simulink model "Exercises_lesson_II"  (R2022b)
settings: Solver=ode23tb  StartTime=0.0  StopTime=10  RelTol=1e-3
values from neighbouring files (symbols this model uses):
  Kb = (ki/kp)    (= 0.25)    [PI_par.m]
  ki = wc * Ri    (= 0.125)    [PI_par.m]
  kp = wc * Li    (= 0.5)    [PI_par.m]
  Li = 0.1    [PI_par.m]
  Ri = 0.025    [PI_par.m]
  sat = 0.3    [PI_par.m]
undefined symbols (not defined in the file or in its folder): sigbuilder_block
libraries: slpidlib x3, spsControlledVoltageSourceLib x1, spsCurrentMeasurementLib x1, spsSeriesRLCBranchLib x1, sps_lib x1
settings Model: Creator=matti  LastModifiedBy=benve
settings SolverCC: AlgebraicLoopSolver=TrustRegion
settings DataIOCC: ReturnWorkspaceOutputs=off
settings DebuggingCC: UnconnectedInputMsg=warning  UnconnectedOutputMsg=warning  UnconnectedLineMsg=warning  SFMachineParentedDataDiag=warning  ArithmeticOperatorsInVariantConditions=warning
settings ModelReferenceCC: EnableRefExpFcnMdlSchedulingChecks=on
settings SFSimCC: SimUseLocalCustomCode=off  CustomCodeUndefinedFunction=UseInterfaceOnly
settings RTWCC: RTWUseLocalCustomCode=off
settings CodeAppCC: StateflowObjectComments=on

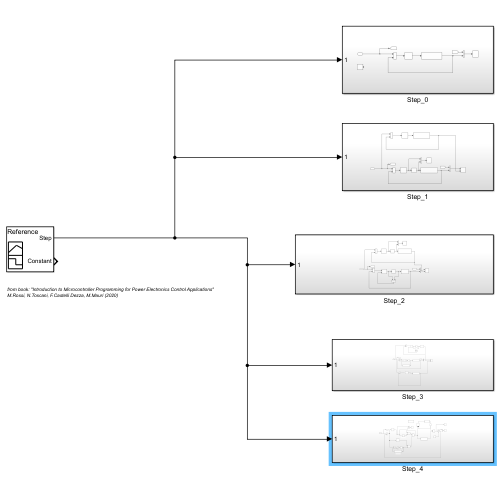
[thumbnail: Simulink's stored preview of the top-level diagram]
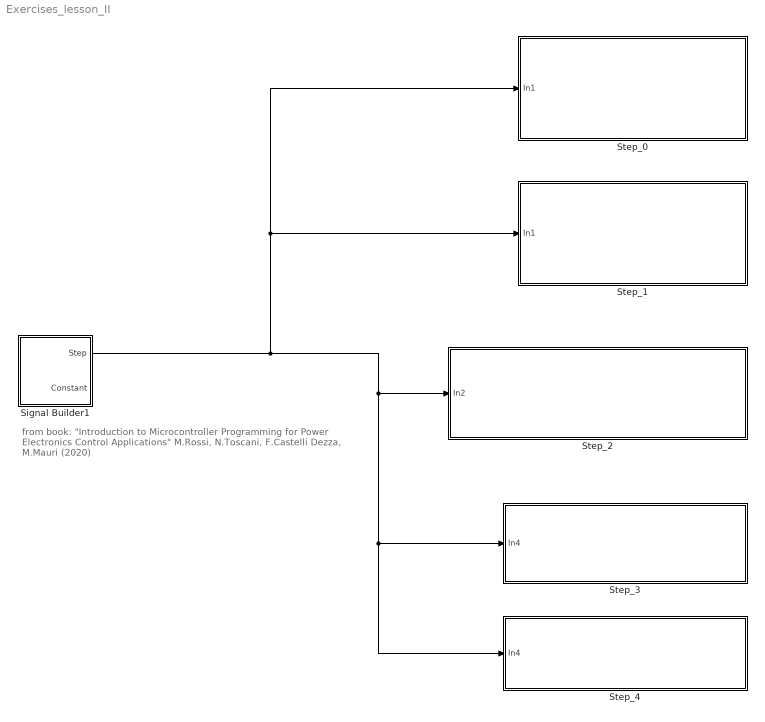
== system Exercises_lesson_II ==
  note: from book: "Introduction to Microcontroller Programming for Power Electronics Control Applications"
      | M.Rossi, N.Toscani, F.Castelli Dezza, M.Mauri (2020)
  Signal Builder1 : Subsystem  Tag=STV Subsys  LoadFcn=sigbuilder_block('load');  StartFcn=sigbuilder_block('start');  StopFcn=sigbuilder_block('stop');  ClipboardFcn=sigbuilder_block('clipboard');  mask(Sigbuilder block){tuvar=[0:10]}
      mask help: Simulink:masks:SigbuilderBlock_MD
      mask init:
      | if ~strcmp(get_param(bdroot(gcbh),'SimulationStatus'),'stopped') tuvar = sigbuilder_block('maskInit'); end
      settings: CopyFcn=sigbuilder_block('copy');  DeleteFcn=sigbuilder_block('delete');  ModelCloseFcn=sigbuilder_block('modelClose');  PreSaveFcn=sigbuilder_block('preSave');  PauseFcn=sigbuilder_block('pause');  ContinueFcn=sigbuilder_block('continue');  NameChangeFcn=sigbuilder_block('namechange');  OpenFcn=sigbuilder_block('open',[5.4 5.4 1141.2 580.8 ]);  CloseFcn=sigbuilder_block('close');
      mask Display: plot(0, 0, 100, 100,[2, 2, 32, 32, 2], [68, 8, 8, 68, 68],[32, 2], [38, 38], [32, 19, 2],[53, 60, 44], [32, 17, 17, 2],[16, 16, 31, 31]);txt = getActiveGroup(gcbh);text(2, 100, txt,'verticalAlignment', 'top');
  Step_0 : Subsystem
  Step_1 : Subsystem
  Step_2 : Subsystem
  Step_3 : Subsystem
  Step_4 : Subsystem
  wires:
  Signal Builder1/1(Step) -> Step_4/1(In4), Step_3/1(In4), Step_2/1(In2), Step_0/1(In1), Step_1/1(In1)

== system Exercises_lesson_II/Signal Builder1 ==
  Demux : Demux  Tag=STV Demux  Outputs=2
      settings: DisplayOption=none
  FromWs : FromWorkspace  Tag=STV FromWs  VariableName=tuvar
      SigBuilderData=|
      | common.afterFinalStr = 'Extrapolate'
      | common.sampleTime = 0
      | dataSet.timeRange = [0 10]
      | dataSet.name = 'Reference'
      | sbobj.Groups.Name = 'Reference'
      | sbobj.Groups.Signals(1).Name = 'Step'
      | sbobj.Groups.Signals(1).XData = [0 1 1 4 4 10]
      | sbobj.Groups.Signals(1).YData = [0 0 1 1 0 0]
      | sbobj.Groups.Signals(2).Name = 'Constant'
      | sbobj.Groups.Signals(2).XData = [0 10]
      | sbobj.Groups.Signals(2).YData = [1 1]
  Step : Outport  Tag=STV Outport
  Constant : Outport  Tag=STV Outport  Port=2
  wires:
  Demux/1 -> Step/1
  FromWs/1 -> Demux/1
  Demux/2 -> Constant/1

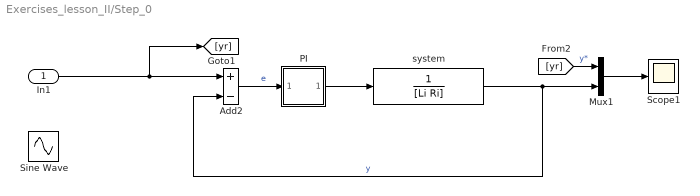
== system Exercises_lesson_II/Step_0 ==
  In1 : Inport
  Add2 : Sum  Inputs=+-
  Mux1 : Mux  Inputs=2
  PI : Subsystem
      mask Display: disp('PI')
  Scope1 : Scope
  Sine Wave : Sin  SampleTime=0
  system : TransferFcn  Denominator=[Li Ri]
  wires:
  [yr] -> Mux1/1  "y*"
  Add2/1 -> PI/1(In1)  "e"
  Mux1/1 -> Scope1/1
  system/1 -> Mux1/2, Add2/2  "y"
  PI/1(Out1) -> system/1
  In1/1 -> [yr], Add2/1

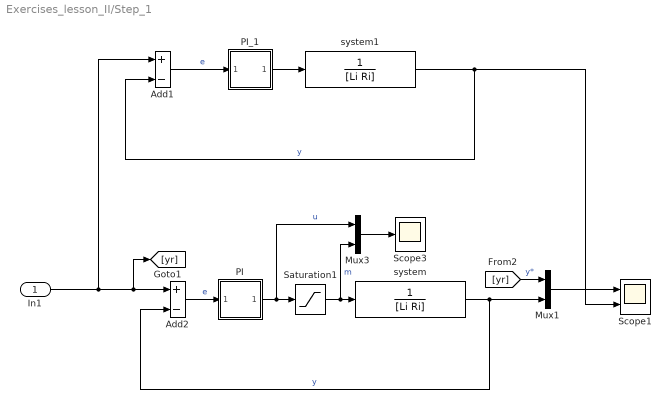
== system Exercises_lesson_II/Step_1 ==
  In1 : Inport
  Add1 : Sum  Inputs=+-
  Add2 : Sum  Inputs=+-
  Mux1 : Mux  Inputs=2
  Mux3 : Mux  Inputs=2
  PI : Subsystem
      mask Display: disp('PI')
  PI_1 : Subsystem
      mask Display: disp('PI')
  Saturation1 : Saturate  UpperLimit=sat  LowerLimit=-sat
  Scope1 : Scope  NumInputPorts=2
  Scope3 : Scope
  system : TransferFcn  Denominator=[Li Ri]
  system1 : TransferFcn  Denominator=[Li Ri]
  wires:
  Mux3/1 -> Scope3/1
  PI/1(Out1) -> Mux3/1, Saturation1/1  "u"
  system/1 -> Add2/2, Mux1/2  "y"
  Mux1/1 -> Scope1/1
  Saturation1/1 -> Mux3/2, system/1  "m"
  Add2/1 -> PI/1(In1)  "e"
  [yr] -> Mux1/1  "y*"
  Add1/1 -> PI_1/1(In1)  "e"
  system1/1 -> Scope1/2, Add1/2  "y"
  In1/1 -> Add1/1, [yr], Add2/1
  PI_1/1(Out1) -> system1/1

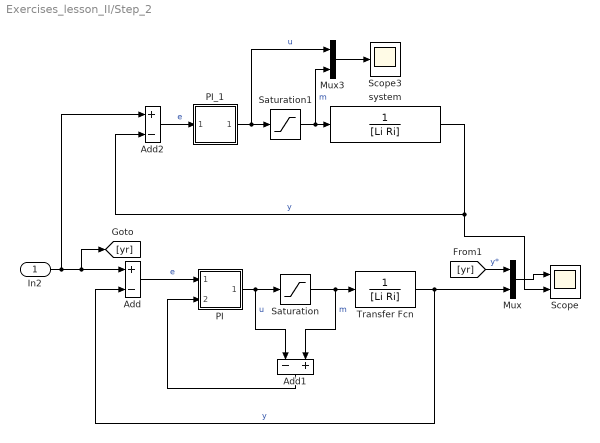
== system Exercises_lesson_II/Step_2 ==
  In2 : Inport
  Add : Sum  Inputs=+-
  Add1 : Sum  Inputs=-+
  Add2 : Sum  Inputs=+-
  Mux : Mux  Inputs=2
  Mux3 : Mux  Inputs=2
  PI : Subsystem
      mask Display: disp('PI')
  PI_1 : Subsystem
      mask Display: disp('PI')
  Saturation : Saturate  UpperLimit=sat  LowerLimit=-sat
  Saturation1 : Saturate  UpperLimit=sat  LowerLimit=-sat
  Scope : Scope  NumInputPorts=2
  Scope3 : Scope
  Transfer Fcn : TransferFcn  Denominator=[Li Ri]
  system : TransferFcn  Denominator=[Li Ri]
  wires:
  Add1/1 -> PI/2(In2)
  PI/1(Out1) -> Add1/1, Saturation/1  "u"
  Saturation/1 -> Add1/2, Transfer Fcn/1  "m"
  Mux/1 -> Scope/1
  Transfer Fcn/1 -> Mux/2, Add/2  "y"
  Add/1 -> PI/1(In1)  "e"
  [yr] -> Mux/1  "y*"
  PI_1/1(Out1) -> Mux3/1, Saturation1/1  "u"
  Add2/1 -> PI_1/1(In1)  "e"
  Mux3/1 -> Scope3/1
  system/1 -> Scope/2, Add2/2  "y"
  In2/1 -> Add2/1, [yr], Add/1
  Saturation1/1 -> Mux3/2, system/1  "m"

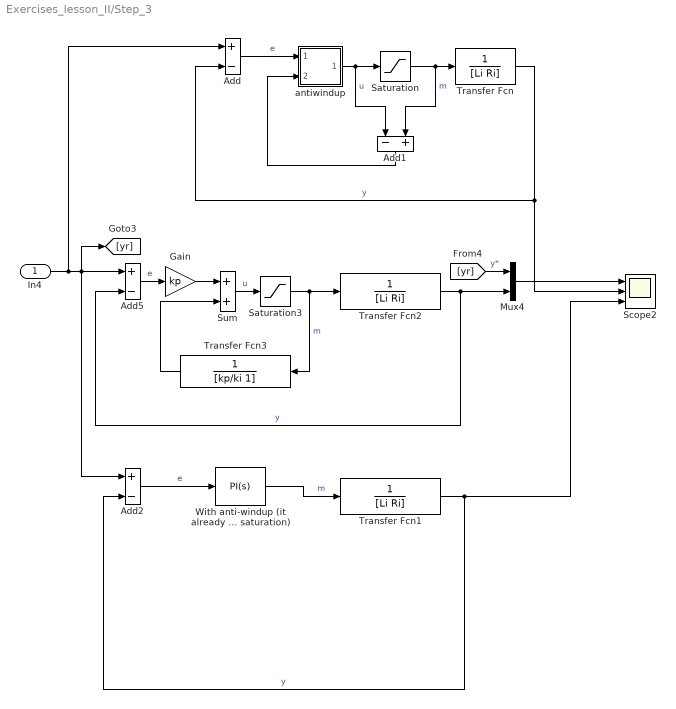
== system Exercises_lesson_II/Step_3 ==
  In4 : Inport
  Add : Sum  Inputs=+-
  Add1 : Sum  Inputs=-+
  Add2 : Sum  Inputs=+-
  Add5 : Sum  Inputs=+-
  Gain : Gain  Gain=kp
  Mux4 : Mux  Inputs=2
  Saturation : Saturate  UpperLimit=sat  LowerLimit=-sat
  Saturation3 : Saturate  UpperLimit=sat  LowerLimit=-sat
  Scope2 : Scope  NumInputPorts=3
  Sum : Sum
  Transfer Fcn : TransferFcn  Denominator=[Li Ri]
  Transfer Fcn1 : TransferFcn  Denominator=[Li Ri]
  Transfer Fcn2 : TransferFcn  Denominator=[Li Ri]
  Transfer Fcn3 : TransferFcn  Denominator=[kp/ki 1]
  With anti-windup (it already considers saturation) : slpidlib/PID Controller  Controller=PI  Form=Parallel  TimeDomain=Continuous-time  UseExternalTs=off  SampleTime=-1  IntegratorMethod=Forward Euler  FilterMethod=Forward Euler  ControllerParametersSource=internal  P=kp  I=ki  UseKiTs=off  D=0  N=100  UseFilter=on  TunerSelectOption=Frequency Response Based  ZeroCross=off  InitialConditionSource=internal  InitialConditionForIntegrator=0  InitialConditionForFilter=0  DifferentiatorICPrevScaledInput=0  ExternalReset=none  TrackingMode=off  Kt=1  LimitOutput=on  SatLimitsSource=internal  UpperSaturationLimit=sat  LowerSaturationLimit=-sat  LinearizeAsGain=on  AntiWindupMode=back-calculation  Kb=Kb  LimitIntegrator=off  UpperIntegratorSaturationLimit=inf  LowerIntegratorSaturationLimit=-inf  POutMin=[]  POutMax=[]  IOutMin=[]  IOutMax=[]  DOutMin=[]  DOutMax=[]  NOutMin=[]  NOutMax=[]  SumOutMin=[]  SumOutMax=[]  SaturationOutMin=[]  SaturationOutMax=[]  PParamMin=[]  PParamMax=[]  IParamMin=[]  IParamMax=[]  DParamMin=[]  DParamMax=[]  NParamMin=[]  NParamMax=[]  KbParamMin=[]  KbParamMax=[]  KtParamMin=[]  KtParamMax=[]  KbOutMin=[]  KbOutMax=[]  KtOutMin=[]  KtOutMax=[]  IntegratorOutMin=[]  IntegratorOutMax=[]  FilterOutMin=[]  FilterOutMax=[]  SumI1OutMin=[]  SumI1OutMax=[]  SumI2OutMin=[]  SumI2OutMax=[]  SumI3OutMin=[]  SumI3OutMax=[]  SumI4OutMin=[]  SumI4OutMax=[]  SumDOutMin=[]  SumDOutMax=[]  DifferentiatorOutMin=[]  DifferentiatorOutMax=[]  FilterDiffOutCoefMin=[]  FilterDiffOutCoefMax=[]  ReciprocalOutMin=[]  ReciprocalOutMax=[]  SumDenOutMin=[]  SumDenOutMax=[]  SumNumOutMin=[]  SumNumOutMax=[]  DivideOutMin=[]  DivideOutMax=[]  UdiffTsProdOutMin=[]  UdiffTsProdOutMax=[]  NTsProdOutMin=[]  NTsProdOutMax=[]  UintegralTsProdOutMin=[]  UintegralTsProdOutMax=[]  UngainTsProdOutMin=[]  UngainTsProdOutMax=[]  ClampingZeroOutDataTypeStr=Inherit: Inherit via back propagation  ClampingZeroOutMin=[]  ClampingZeroOutMax=[]  FilterDenConstantOutDataTypeStr=Inherit: Inherit via back propagation  FilterDenConstantOutMin=[]  FilterDenConstantOutMax=[]  PCopyOutDataTypeStr=Inherit: Inherit via back propagation  PCopyOutMin=[]  PCopyOutMax=[]  NCopyOutDataTypeStr=Inherit: Inherit via back propagation  NCopyOutMin=[]  NCopyOutMax=[]  IntegratorContinuousStateAttributes=''  IntegratorStateMustResolveToSignalObject=off  IntegratorRTWStateStorageClass=Auto  FilterContinuousStateAttributes=''  FilterStateMustResolveToSignalObject=off  FilterRTWStateStorageClass=Auto  ParallelPVariant=InternalParameters  IdealPVariant=Disabled  IVariant=InternalParameters  DVariant=Disabled  IntegratorVariant=Continuous  SatVariant=Enabled  AWVariant=BackCalculation  PCopyVariant=Disabled  TRVariant=Disabled  FdbkBlocksVariant=Forward  IdealPFdbkVariant=Disabled  SatFdbkVariant=Disabled  DerivativeFilterVariant=Disabled  NVariant=Disabled  NCopyVariant=Disabled_SignalSpec  FilterICVariant=Disabled  IntegratorICVariant=InternalICs  ExternalResetVariant=Disabled  TRSumVariant=Passthrough  SumFdbkVariant=Disabled  SumVariant=Sum_PI  TsampFilterVariant=InternalTs  TsampNgainVariant=Passthrough  TsampIntegralVariant=Passthrough  ExternalSaturationOutDataTypeStr=Inherit: Same as second input
  antiwindup : Subsystem
      mask Display: disp('PI')
  wires:
  Mux4/1 -> Scope2/1
  Transfer Fcn2/1 -> Mux4/2, Add5/2  "y"
  [yr] -> Mux4/1  "y*"
  Add5/1 -> Gain/1  "e"
  Gain/1 -> Sum/1
  Saturation3/1 -> Transfer Fcn2/1, Transfer Fcn3/1  "m"
  Transfer Fcn3/1 -> Sum/2
  Sum/1 -> Saturation3/1  "u"
  Saturation/1 -> Add1/2, Transfer Fcn/1  "m"
  Transfer Fcn/1 -> Scope2/2, Add/2  "y"
  Add/1 -> antiwindup/1(In1)  "e"
  antiwindup/1(Out1) -> Add1/1, Saturation/1  "u"
  Add1/1 -> antiwindup/2(In2)
  In4/1 -> Add2/1, [yr], Add5/1, Add/1
  Add2/1 -> With anti-windup (it already considers saturation)/1  "e"
  Transfer Fcn1/1 -> Scope2/3, Add2/2  "y"
  With anti-windup (it already considers saturation)/1 -> Transfer Fcn1/1  "m"

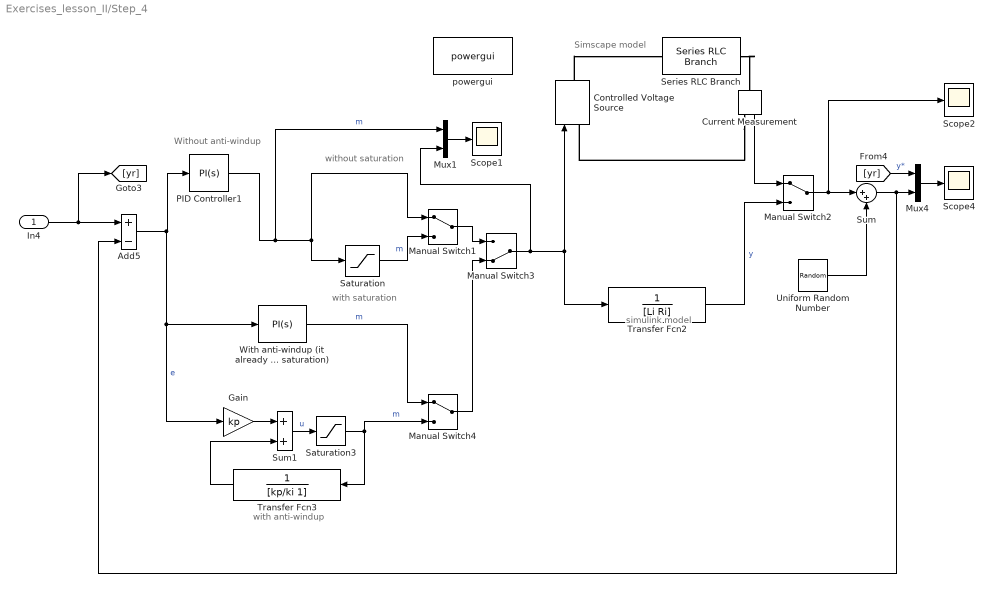
== system Exercises_lesson_II/Step_4 ==
  note: with anti-windup
  note: simulink model
  note: with saturation
  note: without saturation
  note: Without anti-windup
  note: Simscape model
  In4 : Inport
  Add5 : Sum  Inputs=+-
  Controlled Voltage Source : spsControlledVoltageSourceLib/Controlled Voltage Source  Initialize=on  Source_Type=AC  Amplitude=0  Phase=0  Frequency=0  Measurements=None
  Current Measurement : spsCurrentMeasurementLib/Current Measurement  PhasorSimulation=off  OutputType=Complex  PSBequivalent=0
  Gain : Gain  Gain=kp
  Manual Switch1 : ManualSwitch
  Manual Switch2 : ManualSwitch
  Manual Switch3 : ManualSwitch  CurrentSetting=0
  Manual Switch4 : ManualSwitch
  Mux1 : Mux  Inputs=2
  Mux4 : Mux  Inputs=2
  PID Controller1 : slpidlib/PID Controller  Controller=PI  Form=Parallel  TimeDomain=Continuous-time  UseExternalTs=off  SampleTime=-1  IntegratorMethod=Forward Euler  FilterMethod=Forward Euler  ControllerParametersSource=internal  P=kp  I=ki  UseKiTs=off  D=0  N=100  UseFilter=on  TunerSelectOption=Transfer Function Based (PID Tuner App)  InitialConditionSource=internal  InitialConditionForIntegrator=0  InitialConditionForFilter=0  DifferentiatorICPrevScaledInput=0  ExternalReset=none  TrackingMode=off  Kt=1  LimitOutput=off  SatLimitsSource=internal  UpperSaturationLimit=sat  LowerSaturationLimit=-sat  LinearizeAsGain=on  AntiWindupMode=none  Kb=Kb  LimitIntegrator=off  UpperIntegratorSaturationLimit=inf  LowerIntegratorSaturationLimit=-inf  POutMin=[]  POutMax=[]  IOutMin=[]  IOutMax=[]  DOutMin=[]  DOutMax=[]  NOutMin=[]  NOutMax=[]  SumOutMin=[]  SumOutMax=[]  SaturationOutMin=[]  SaturationOutMax=[]  PParamMin=[]  PParamMax=[]  IParamMin=[]  IParamMax=[]  DParamMin=[]  DParamMax=[]  NParamMin=[]  NParamMax=[]  KbParamMin=[]  KbParamMax=[]  KtParamMin=[]  KtParamMax=[]  KbOutMin=[]  KbOutMax=[]  KtOutMin=[]  KtOutMax=[]  IntegratorOutMin=[]  IntegratorOutMax=[]  FilterOutMin=[]  FilterOutMax=[]  SumI1OutMin=[]  SumI1OutMax=[]  SumI2OutMin=[]  SumI2OutMax=[]  SumI3OutMin=[]  SumI3OutMax=[]  SumI4OutMin=[]  SumI4OutMax=[]  SumDOutMin=[]  SumDOutMax=[]  DifferentiatorOutMin=[]  DifferentiatorOutMax=[]  FilterDiffOutCoefMin=[]  FilterDiffOutCoefMax=[]  ReciprocalOutMin=[]  ReciprocalOutMax=[]  SumDenOutMin=[]  SumDenOutMax=[]  SumNumOutMin=[]  SumNumOutMax=[]  DivideOutMin=[]  DivideOutMax=[]  UdiffTsProdOutMin=[]  UdiffTsProdOutMax=[]  NTsProdOutMin=[]  NTsProdOutMax=[]  UintegralTsProdOutMin=[]  UintegralTsProdOutMax=[]  UngainTsProdOutMin=[]  UngainTsProdOutMax=[]  ClampingZeroOutDataTypeStr=Inherit: Inherit via back propagation  ClampingZeroOutMin=[]  ClampingZeroOutMax=[]  FilterDenConstantOutDataTypeStr=Inherit: Inherit via back propagation  FilterDenConstantOutMin=[]  FilterDenConstantOutMax=[]  PCopyOutDataTypeStr=Inherit: Inherit via back propagation  PCopyOutMin=[]  PCopyOutMax=[]  NCopyOutDataTypeStr=Inherit: Inherit via back propagation  NCopyOutMin=[]  NCopyOutMax=[]  IntegratorContinuousStateAttributes=''  IntegratorStateMustResolveToSignalObject=off  IntegratorRTWStateStorageClass=Auto  FilterContinuousStateAttributes=''  FilterStateMustResolveToSignalObject=off  FilterRTWStateStorageClass=Auto  ParallelPVariant=InternalParameters  IdealPVariant=Disabled  IVariant=InternalParameters  DVariant=Disabled  IntegratorVariant=Continuous  SatVariant=Disabled  AWVariant=Passthrough  PCopyVariant=Disabled  TRVariant=Disabled  FdbkBlocksVariant=Forward  IdealPFdbkVariant=Disabled  SatFdbkVariant=Disabled  DerivativeFilterVariant=Disabled  NVariant=Disabled  NCopyVariant=Disabled_SignalSpec  FilterICVariant=Disabled  IntegratorICVariant=InternalICs  ExternalResetVariant=Disabled  TRSumVariant=Passthrough  SumFdbkVariant=Disabled  SumVariant=Sum_PI  TsampFilterVariant=InternalTs  TsampNgainVariant=Passthrough  TsampIntegralVariant=Passthrough  ExternalSaturationOutDataTypeStr=Inherit: Same as second input
  Saturation : Saturate  UpperLimit=sat  LowerLimit=-sat
  Saturation3 : Saturate  UpperLimit=sat  LowerLimit=-sat
  Scope1 : Scope
  Scope2 : Scope
  Scope4 : Scope
  Series RLC Branch : spsSeriesRLCBranchLib/Series RLC Branch  LConnTagsString=__new0  RConnTagsString=__new0  BranchType=RL  Resistance=Ri  Inductance=Li  SetiL0=off  InitialCurrent=0  Capacitance=1e-6  Setx0=off  InitialVoltage=0  Measurements=None
  Sum : Sum  Inputs=|++
  Sum1 : Sum
  Transfer Fcn2 : TransferFcn  Denominator=[Li Ri]
  Transfer Fcn3 : TransferFcn  Denominator=[kp/ki 1]
  Uniform Random Number : UniformRandomNumber  Minimum=-0.05  Maximum=0.05  SampleTime=0.1
  With anti-windup (it already considers saturation) : slpidlib/PID Controller  Controller=PI  Form=Parallel  TimeDomain=Continuous-time  UseExternalTs=off  SampleTime=-1  IntegratorMethod=Forward Euler  FilterMethod=Forward Euler  ControllerParametersSource=internal  P=kp  I=ki  UseKiTs=off  D=0  N=100  UseFilter=on  TunerSelectOption=Frequency Response Based  ZeroCross=off  InitialConditionSource=internal  InitialConditionForIntegrator=0  InitialConditionForFilter=0  DifferentiatorICPrevScaledInput=0  ExternalReset=none  TrackingMode=off  Kt=1  LimitOutput=on  SatLimitsSource=internal  UpperSaturationLimit=sat  LowerSaturationLimit=-sat  LinearizeAsGain=on  AntiWindupMode=back-calculation  Kb=Kb  LimitIntegrator=off  UpperIntegratorSaturationLimit=inf  LowerIntegratorSaturationLimit=-inf  POutMin=[]  POutMax=[]  IOutMin=[]  IOutMax=[]  DOutMin=[]  DOutMax=[]  NOutMin=[]  NOutMax=[]  SumOutMin=[]  SumOutMax=[]  SaturationOutMin=[]  SaturationOutMax=[]  PParamMin=[]  PParamMax=[]  IParamMin=[]  IParamMax=[]  DParamMin=[]  DParamMax=[]  NParamMin=[]  NParamMax=[]  KbParamMin=[]  KbParamMax=[]  KtParamMin=[]  KtParamMax=[]  KbOutMin=[]  KbOutMax=[]  KtOutMin=[]  KtOutMax=[]  IntegratorOutMin=[]  IntegratorOutMax=[]  FilterOutMin=[]  FilterOutMax=[]  SumI1OutMin=[]  SumI1OutMax=[]  SumI2OutMin=[]  SumI2OutMax=[]  SumI3OutMin=[]  SumI3OutMax=[]  SumI4OutMin=[]  SumI4OutMax=[]  SumDOutMin=[]  SumDOutMax=[]  DifferentiatorOutMin=[]  DifferentiatorOutMax=[]  FilterDiffOutCoefMin=[]  FilterDiffOutCoefMax=[]  ReciprocalOutMin=[]  ReciprocalOutMax=[]  SumDenOutMin=[]  SumDenOutMax=[]  SumNumOutMin=[]  SumNumOutMax=[]  DivideOutMin=[]  DivideOutMax=[]  UdiffTsProdOutMin=[]  UdiffTsProdOutMax=[]  NTsProdOutMin=[]  NTsProdOutMax=[]  UintegralTsProdOutMin=[]  UintegralTsProdOutMax=[]  UngainTsProdOutMin=[]  UngainTsProdOutMax=[]  ClampingZeroOutDataTypeStr=Inherit: Inherit via back propagation  ClampingZeroOutMin=[]  ClampingZeroOutMax=[]  FilterDenConstantOutDataTypeStr=Inherit: Inherit via back propagation  FilterDenConstantOutMin=[]  FilterDenConstantOutMax=[]  PCopyOutDataTypeStr=Inherit: Inherit via back propagation  PCopyOutMin=[]  PCopyOutMax=[]  NCopyOutDataTypeStr=Inherit: Inherit via back propagation  NCopyOutMin=[]  NCopyOutMax=[]  IntegratorContinuousStateAttributes=''  IntegratorStateMustResolveToSignalObject=off  IntegratorRTWStateStorageClass=Auto  FilterContinuousStateAttributes=''  FilterStateMustResolveToSignalObject=off  FilterRTWStateStorageClass=Auto  ParallelPVariant=InternalParameters  IdealPVariant=Disabled  IVariant=InternalParameters  DVariant=Disabled  IntegratorVariant=Continuous  SatVariant=Enabled  AWVariant=BackCalculation  PCopyVariant=Disabled  TRVariant=Disabled  FdbkBlocksVariant=Forward  IdealPFdbkVariant=Disabled  SatFdbkVariant=Disabled  DerivativeFilterVariant=Disabled  NVariant=Disabled  NCopyVariant=Disabled_SignalSpec  FilterICVariant=Disabled  IntegratorICVariant=InternalICs  ExternalResetVariant=Disabled  TRSumVariant=Passthrough  SumFdbkVariant=Disabled  SumVariant=Sum_PI  TsampFilterVariant=InternalTs  TsampNgainVariant=Passthrough  TsampIntegralVariant=Passthrough  ExternalSaturationOutDataTypeStr=Inherit: Same as second input
  powergui : sps_lib/powergui  Priority=1  SimulationMode=Continuous  SampleTime=50e-6  frequency=60  Iterations=50  frequencyindice=0  Pbase=100e6  ErrMax=1e-4  UnitsV=kV  UnitsW=MW  buscounter=0  FunctionMessages=off  echomessages=off  EnableUseOfTLC=off  CurrentSourceSwitches=off  DisableSnubberDevices=off  DisableRonSwitches=off  DisableVfSwitches=off  DisplayEquations=off  AutomaticDiscreteSolvers=off  SolverType=Tustin/Backward Euler (TBE)  Interpol=off  ExternalGateDelay=off  methode=off  Ts=100  x0status=blocks  SPID=on  SwTol=0  HookPort=off  NonlinearTolerance=1e-4  nMaxIteration=100  ContinueOnMaxIteration=off  RestoreLinks=warning  ResistiveCurrentMeasurement=off  Frange=[0:2:500]  Ylog=off  Xlog=on  ShowGrid=off  save=off  variable=ZData  structure=0  ZoomFFT=off  StartTime=0.0  cycles=1  DisplayStyle=1  fundamental=60  FreqAxis=off  MaxFrequency=1000  frequencyindicesteady=1  RmsSteady=1  display=off
  wires:
  In4/1 -> Add5/1, [yr]
  [yr] -> Mux4/1  "y*"
  Transfer Fcn2/1 -> Manual Switch2/2  "y"
  Mux4/1 -> Scope4/1
  Saturation/1 -> Manual Switch1/2  "m"
  Current Measurement/1 -> Manual Switch2/1
  Manual Switch2/1 -> Scope2/1, Sum/1
  PID Controller1/1 -> Mux1/1, Manual Switch1/1, Saturation/1  "m"
  With anti-windup (it already considers saturation)/1 -> Manual Switch4/1  "m"
  Manual Switch1/1 -> Manual Switch3/1
  Manual Switch3/1 -> Mux1/2, Controlled Voltage Source/1, Transfer Fcn2/1
  Sum/1 -> Mux4/2, Add5/2
  Mux1/1 -> Scope1/1
  Saturation3/1 -> Manual Switch4/2, Transfer Fcn3/1  "m"
  Transfer Fcn3/1 -> Sum1/2
  Sum1/1 -> Saturation3/1  "u"
  Add5/1 -> Gain/1, With anti-windup (it already considers saturation)/1, PID Controller1/1  "e"
  Gain/1 -> Sum1/1
  Manual Switch4/1 -> Manual Switch3/2
  Uniform Random Number/1 -> Sum/2
  connections:
  Controlled Voltage Source/RConn1 -- Series RLC Branch/LConn1
  Series RLC Branch/RConn1 -- Current Measurement/LConn1
  Current Measurement/RConn1 -- Controlled Voltage Source/LConn1

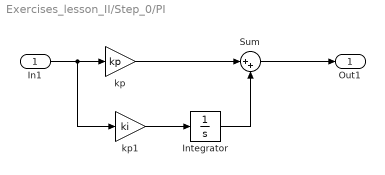
== system Exercises_lesson_II/Step_0/PI ==
  In1 : Inport
  Integrator : Integrator
  Sum : Sum  Inputs=|++
  kp : Gain  Gain=kp
  kp1 : Gain  Gain=ki
  Out1 : Outport  VectorParamsAs1DForOutWhenUnconnected=off
  wires:
  kp1/1 -> Integrator/1
  In1/1 -> kp1/1, kp/1
  Integrator/1 -> Sum/2
  kp/1 -> Sum/1
  Sum/1 -> Out1/1

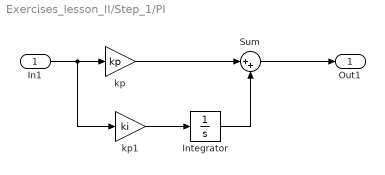
== system Exercises_lesson_II/Step_1/PI ==
  In1 : Inport
  Integrator : Integrator
  Sum : Sum  Inputs=|++
  kp : Gain  Gain=kp
  kp1 : Gain  Gain=ki
  Out1 : Outport  VectorParamsAs1DForOutWhenUnconnected=off
  wires:
  kp1/1 -> Integrator/1
  In1/1 -> kp1/1, kp/1
  Integrator/1 -> Sum/2
  kp/1 -> Sum/1
  Sum/1 -> Out1/1

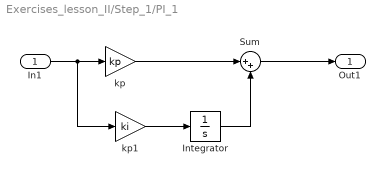
== system Exercises_lesson_II/Step_1/PI_1 ==
  In1 : Inport
  Integrator : Integrator
  Sum : Sum  Inputs=|++
  kp : Gain  Gain=kp
  kp1 : Gain  Gain=ki
  Out1 : Outport  VectorParamsAs1DForOutWhenUnconnected=off
  wires:
  kp1/1 -> Integrator/1
  In1/1 -> kp1/1, kp/1
  Integrator/1 -> Sum/2
  kp/1 -> Sum/1
  Sum/1 -> Out1/1

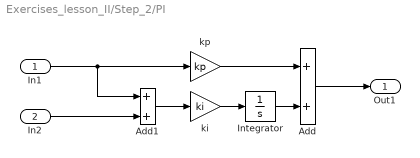
== system Exercises_lesson_II/Step_2/PI ==
  In1 : Inport
  In2 : Inport  Port=2
  Add : Sum
  Add1 : Sum
  Integrator : Integrator
  ki : Gain  Gain=ki
  kp : Gain  Gain=kp
  Out1 : Outport  VectorParamsAs1DForOutWhenUnconnected=off
  wires:
  Integrator/1 -> Add/2
  ki/1 -> Integrator/1
  kp/1 -> Add/1
  In1/1 -> kp/1, Add1/1
  Add/1 -> Out1/1
  Add1/1 -> ki/1
  In2/1 -> Add1/2

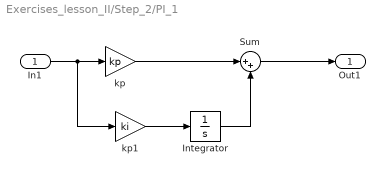
== system Exercises_lesson_II/Step_2/PI_1 ==
  In1 : Inport
  Integrator : Integrator
  Sum : Sum  Inputs=|++
  kp : Gain  Gain=kp
  kp1 : Gain  Gain=ki
  Out1 : Outport  VectorParamsAs1DForOutWhenUnconnected=off
  wires:
  kp1/1 -> Integrator/1
  In1/1 -> kp1/1, kp/1
  Integrator/1 -> Sum/2
  kp/1 -> Sum/1
  Sum/1 -> Out1/1

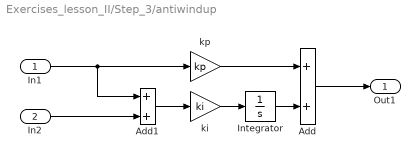
== system Exercises_lesson_II/Step_3/antiwindup ==
  In1 : Inport
  In2 : Inport  Port=2
  Add : Sum
  Add1 : Sum
  Integrator : Integrator
  ki : Gain  Gain=ki
  kp : Gain  Gain=kp
  Out1 : Outport  VectorParamsAs1DForOutWhenUnconnected=off
  wires:
  Integrator/1 -> Add/2
  ki/1 -> Integrator/1
  kp/1 -> Add/1
  In1/1 -> kp/1, Add1/1
  Add/1 -> Out1/1
  Add1/1 -> ki/1
  In2/1 -> Add1/2
